simulink model "Sim_MyFirst"  (R2022a)
settings: Solver=ode4  StartTime=0.0  StopTime=t_end  FixedStep=0.0002  RelTol=1e-3  EnableMultiTasking=on
values from neighbouring files (symbols this model uses):
  den_Cfb = [0.00109873559912302  1  0]    [main.m]
  denominator_P = [mass 0 0]    [main.m]
  num_Cfb = [179824.76349148  33696607.3425078  876981355.154548]    [main.m]
  numerator_P = [1]    [main.m]
settings Model: Creator=JC  LastModifiedBy=JC
settings DataIOCC: ReturnWorkspaceOutputs=off

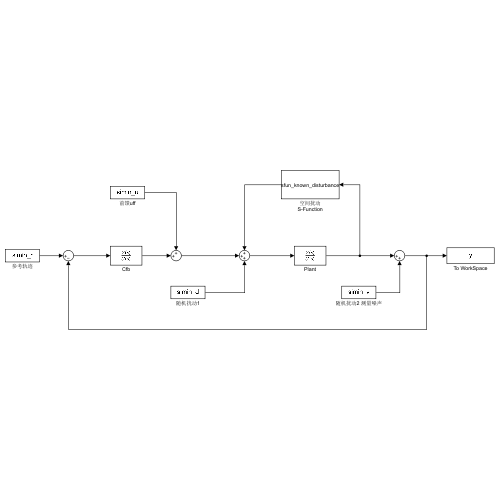
[thumbnail: Simulink's stored preview of the top-level diagram]
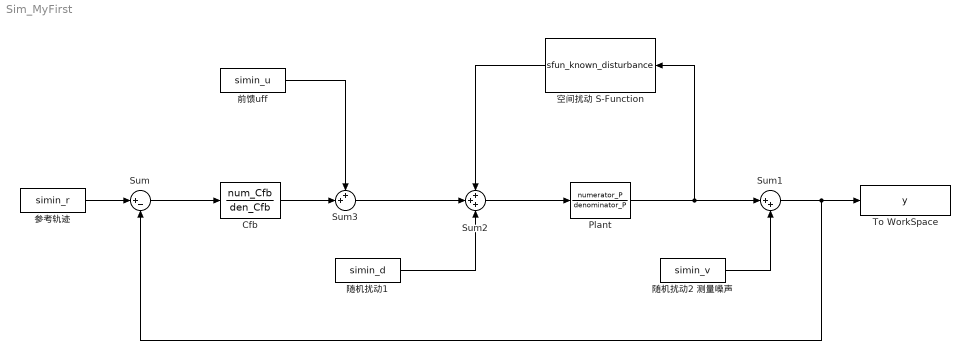
== system Sim_MyFirst ==
  Cfb : TransferFcn  Numerator=num_Cfb  Denominator=den_Cfb
  Plant : TransferFcn  Numerator=numerator_P  Denominator=denominator_P
  Sum : Sum  Inputs=|+-
  Sum1 : Sum  Inputs=|++
  Sum2 : Sum  Inputs=+++
  Sum3 : Sum  Inputs=++|
  To WorkSpace : ToWorkspace  VariableName=y  SampleTime=-1
  前馈uff : FromWorkspace  VariableName=simin_u
  参考轨迹 : FromWorkspace  VariableName=simin_r
  空间扰动 S-Function : S-Function  FunctionName=sfun_known_disturbance  SFunctionDeploymentMode=off  EnableBusSupport=off
  随机扰动1 : FromWorkspace  VariableName=simin_d
  随机扰动2 测量噪声 : FromWorkspace  VariableName=simin_v
  wires:
  Plant/1 -> 空间扰动 S-Function/1, Sum1/1
  随机扰动2 测量噪声/1 -> Sum1/2
  Sum1/1 -> Sum/2, To WorkSpace/1
  Sum2/1 -> Plant/1
  空间扰动 S-Function/1 -> Sum2/1
  Sum/1 -> Cfb/1
  Cfb/1 -> Sum3/2
  Sum3/1 -> Sum2/2
  随机扰动1/1 -> Sum2/3
  前馈uff/1 -> Sum3/1
  参考轨迹/1 -> Sum/1
